simulink model "calcThresholds"  (R2012b)
settings: Solver=FixedStepDiscrete  StartTime=0.0  StopTime=10.0  FixedStep=0.001  RelTol=1e-3
settings Model: BufferReuse=off  Creator=gilja  LastModifiedBy=Chethan
settings SolverCC: EnableConcurrentExecution=on  ConcurrentTasks=on
settings DataIOCC: SaveOutput=off  SignalLogging=off  DSMLogging=off  SaveTime=off
settings OptimizationCC: InlineParams=on  InlineInvariantSignals=on  OptimizeBlockIOStorage=off  BufferReuse=off  ExpressionFolding=off  LocalBlockOutputs=off  SimCompilerOptimization=On
settings HardwareCC: ProdIntDivRoundTo=Zero  ProdEndianess=LittleEndian  ProdHWDeviceType=Generic->32-bit x86 compatible
settings ModelReferenceCC: ModelReferenceMinAlgLoopOccurrences=on
settings RTWCC: SystemTargetFile=xpctarget.tlc  TemplateMakefile=xpc_default_tmf  Description=xPC Target  ProcessScript=xpctarget_make_rtw_hook  RTWCompilerOptimization=On
settings CodeAppCC: MaxIdLength=62
settings xpcTargetCC: TargetFcnLib=ansi_tfl_table_tmw.mat  CodeReplacementLibrary=XPC_BLAS  ParMdlRefBuildCompliant=on  ConcurrentExecutionCompliant=on  CombineSignalStateStructs=off  GRTInterface=on  xPCTaskExecutionProfile=on  xPCRL32EventNumber=5000  xPCisDownloadable=off  xPCLoadParamSetFile=off  xPCConcurrentTasks=off  xPCEnableSFAnimation=off

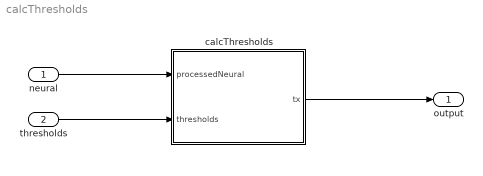
== system calcThresholds ==
  neural : Inport  OutDataTypeStr=Bus: processedNeural
  thresholds : Inport  Port=2
  calcThresholds : MATLAB Function  TreatAsAtomicUnit=on
  output : Outport  BusOutputAsStruct=on
  wires:
  calcThresholds/1(tx) -> output/1
  neural/1 -> calcThresholds/1(processedNeural)
  thresholds/1 -> calcThresholds/2(thresholds)

== matlab function calcThresholds/calcThresholds ==
  data: tx output; processedNeural input Bus: processedNeural; thresholds input double size=[double(DecoderConstants.NUM_CHANNELS_PER_ARRAY) 1]
function tx = calcThresholds(processedNeural, thresholds)
    persistent txOut
    if isempty(txOut)
        txOut = double(zeros(size(processedNeural.minSpikeBand)));
    end

    for x = coder.unroll(1:uint16(DecoderConstants.NUM_CHANNELS_PER_ARRAY))
        thresh = thresholds(x);
        if thresh < 0
            txOut(x) = double(processedNeural.minSpikeBand(x) < thresh);
        else
            txOut(x) = double(processedNeural.maxSpikeBand(x) > thresh);
        end
    end
    
    tx = txOut;
